simulink subsystem "Controlador_evita"  (R2023b)
settings: Solver=VariableStepAuto  StartTime=0.0  StopTime=10.0  RelTol=1e-3
libraries: simulink x2
settings Model: Creator=alumnos  LastModifiedBy=alumnos

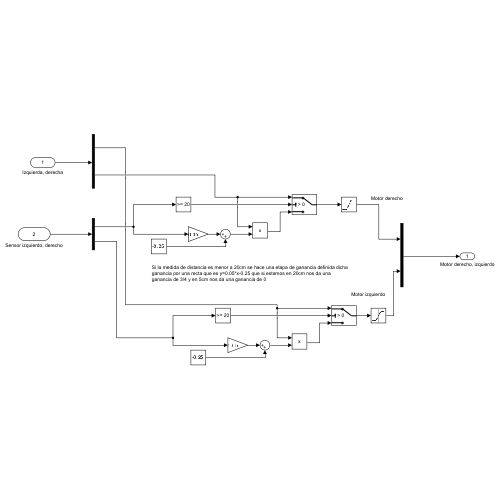
[thumbnail: Simulink's stored preview of the top-level diagram]
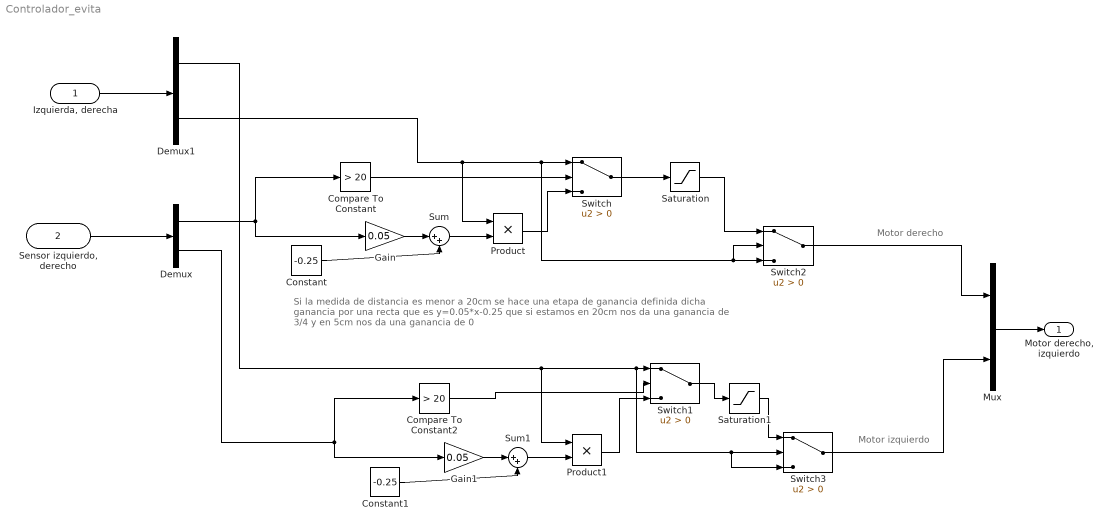
== system Controlador_evita ==
  note: Si la medida de distancia es menor a 20cm se hace una etapa de ganancia definida dicha ganancia por una recta que es y=0.05*x-0.25 que si estamos en 20cm nos da una ganancia de 3/4 y en 5cm nos da una ganancia de 0
  note: Motor izquierdo
  note: Motor derecho
  "Izquierda, derecha" : Inport
  "Sensor izquierdo, derecho" : Inport  Port=2
  Compare To Constant : simulink/Logic and Bit Operations/Compare To Constant  relop=>  const=20  OutDataTypeStr=boolean
  Compare To Constant2 : simulink/Logic and Bit Operations/Compare To Constant  relop=>  const=20  OutDataTypeStr=boolean
  Constant : Constant  Value=-0.25
  Constant1 : Constant  Value=-0.25
  Demux : Demux  Outputs=2
  Demux1 : Demux  Outputs=2
  Gain : Gain  Gain=0.05
  Gain1 : Gain  Gain=0.05
  Mux : Mux  Inputs=2
  Product : Product
  Product1 : Product
  Saturation : Saturate  UpperLimit=255  LowerLimit=0
  Saturation1 : Saturate  UpperLimit=255  LowerLimit=0
  Sum : Sum  Inputs=|++
  Sum1 : Sum  Inputs=|++
  Switch{,1..3} (4 alike) : Switch  Criteria=u2 > Threshold  SaturateOnIntegerOverflow=off  InputSameDT=off
  "Motor derecho, izquierdo" : Outport
  wires:
  "Sensor izquierdo, derecho"/1 -> Demux/1
  Demux/1 -> Gain/1, Compare To Constant/1
  Compare To Constant/1 -> Switch/2
  "Izquierda, derecha"/1 -> Demux1/1
  Demux1/2 -> Product/1, Switch/1, Switch2/3, Switch2/2
  Gain/1 -> Sum/1
  Constant/1 -> Sum/2
  Switch/1 -> Saturation/1
  Sum/1 -> Product/2
  Product/1 -> Switch/3
  Mux/1 -> "Motor derecho, izquierdo"/1
  Compare To Constant2/1 -> Switch1/2
  Demux/2 -> Gain1/1, Compare To Constant2/1
  Switch1/1 -> Saturation1/1
  Sum1/1 -> Product1/2
  Gain1/1 -> Sum1/1
  Constant1/1 -> Sum1/2
  Demux1/1 -> Switch1/1, Switch3/2, Switch3/3, Product1/1
  Product1/1 -> Switch1/3
  Saturation1/1 -> Switch3/1
  Switch3/1 -> Mux/2
  Saturation/1 -> Switch2/1
  Switch2/1 -> Mux/1
